simulink model "parrot_communication_host"  (R2024b)
settings: Solver=FixedStepAuto  StartTime=0.0  StopTime=inf  FixedStep=0.05  RelTol=1e-3
undefined symbols (not defined in the file or in its folder): f
libraries: instrumentlib x7
settings Model: ExtModeTrigDuration=80  Creator=The MathWorks, Inc.  LastModifiedBy=28029
settings SolverCC: AlgebraicLoopSolver=TrustRegion
settings DataIOCC: ReturnWorkspaceOutputs=off
settings OptimizationCC: DefaultParameterBehavior=Inlined  EnhancedBackFolding=on  PassReuseOutputArgsAs=Individual arguments  MaxStackSize=64  OptimizeBlockOrder=speed  DifferentSizesBufferReuse=on  OptimizationCustomize=off  EfficientTunableParamExpr=on
settings DebuggingCC: ParameterTunabilityLossMsg=error  UnconnectedInputMsg=warning  UnconnectedOutputMsg=warning  UnconnectedLineMsg=warning  ArithmeticOperatorsInVariantConditions=warning
settings HardwareCC: ProdBitPerPointer=32  ProdBitPerSizeT=32  ProdBitPerPtrDiffT=32  ProdLargestAtomicInteger=Long  ProdWordSize=32  ProdHWDeviceType=ARM Compatible->ARM 9  UseEmbeddedCoderFeatures=off  UseSimulinkCoderFeatures=off
settings ModelReferenceCC: EnableRefExpFcnMdlSchedulingChecks=on
settings SFSimCC: SimUseLocalCustomCode=off  MATLABDynamicMemAlloc=off  CustomCodeUndefinedFunction=UseInterfaceOnly
settings RTWCC: Description=Embedded Coder  SystemTargetFile=ert.tlc  TemplateMakefile=ert_default_tmf  GenerateReport=on  RTWUseLocalCustomCode=off  Toolchain=Sourcery G++ Lite GNU Toolchain for Drones  IncludeHyperlinkInReport=on  LaunchReport=on  GenerateTraceInfo=on  GenerateTraceReport=on  GenerateTraceReportSl=on  GenerateTraceReportSf=on  GenerateTraceReportEml=on  GPUComputeCapability=3.5
settings CodeAppCC: ForceParamTrailComments=on  IgnoreCustomStorageClasses=off  OperatorAnnotations=on  SimulinkDataObjDesc=on  SFDataObjDesc=on  InsertBlockDesc=on
settings ERTTargetCC: ERTCustomFileTemplate=example_file_process.tlc  DynamicArrayContainerType=coder::array

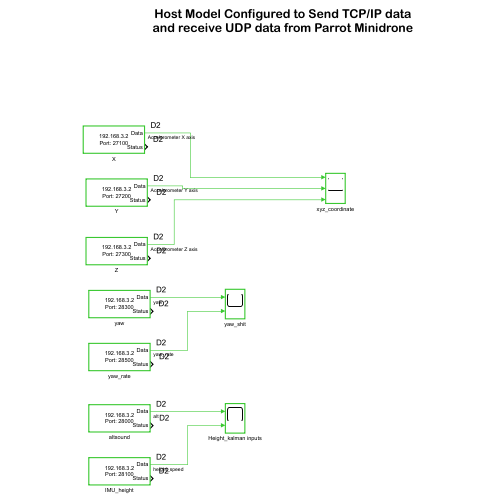
[thumbnail: Simulink's stored preview of the top-level diagram]
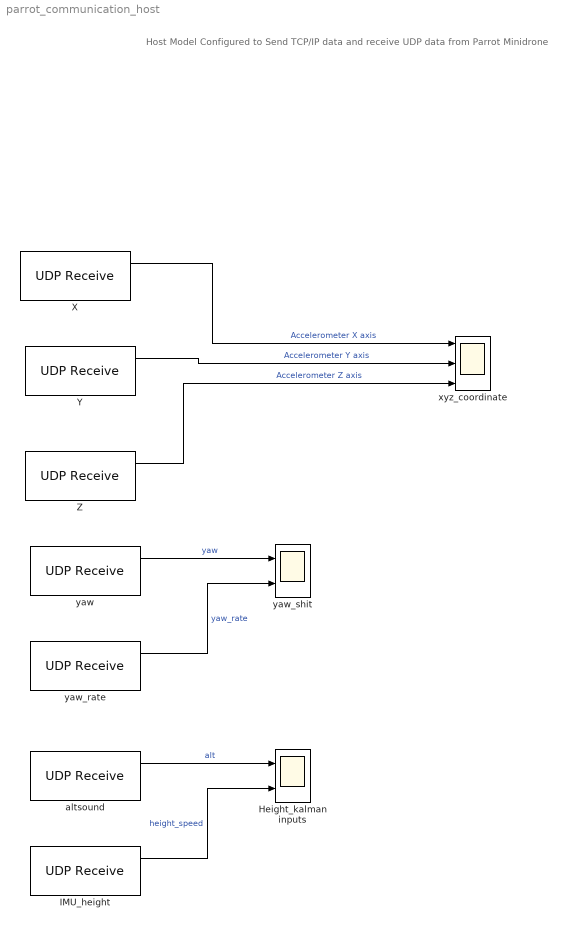
== system parrot_communication_host ==
  note: Host Model Configured to Send TCP/IP data
      | and receive UDP data from Parrot Minidrone
  Height_kalman inputs : Scope  NumInputPorts=2
  IMU_height : instrumentlib/UDP Receive  LocalAddress=192.168.3.2  LocalPort=28100  EnablePortSharing=off  Host=192.168.3.5  Port=29000  GetLatestData=off  DataSize=1  DataType=single  ASCIIFormatting=%f,  Terminator=LF  CustomTerminator=10  ByteOrder=little-endian  EnableBlockingMode=off  Timeout=10  SampleTime=1  SimulateUsing=Interpreted execution
  X : instrumentlib/UDP Receive  LocalAddress=192.168.3.2  LocalPort=27100  EnablePortSharing=off  Host=192.168.3.5  Port=29000  GetLatestData=off  DataSize=1  DataType=single  ASCIIFormatting=%f,  Terminator=LF  CustomTerminator=10  ByteOrder=little-endian  EnableBlockingMode=off  Timeout=10  SampleTime=1  SimulateUsing=Interpreted execution
  Y : instrumentlib/UDP Receive  LocalAddress=192.168.3.2  LocalPort=27200  EnablePortSharing=off  Host=192.168.3.5  Port=29000  GetLatestData=off  DataSize=1  DataType=single  ASCIIFormatting=%f,  Terminator=LF  CustomTerminator=10  ByteOrder=little-endian  EnableBlockingMode=off  Timeout=10  SampleTime=1  SimulateUsing=Interpreted execution
  Z : instrumentlib/UDP Receive  LocalAddress=192.168.3.2  LocalPort=27300  EnablePortSharing=off  Host=192.168.3.5  Port=29000  GetLatestData=off  DataSize=1  DataType=single  ASCIIFormatting=%f,  Terminator=LF  CustomTerminator=10  ByteOrder=little-endian  EnableBlockingMode=off  Timeout=10  SampleTime=1  SimulateUsing=Interpreted execution
  altsound : instrumentlib/UDP Receive  LocalAddress=192.168.3.2  LocalPort=28000  EnablePortSharing=off  Host=192.168.3.5  Port=29000  GetLatestData=off  DataSize=1  DataType=single  ASCIIFormatting=%f,  Terminator=LF  CustomTerminator=10  ByteOrder=little-endian  EnableBlockingMode=off  Timeout=10  SampleTime=1  SimulateUsing=Interpreted execution
  xyz_coordinate : Scope  NumInputPorts=3
  yaw : instrumentlib/UDP Receive  LocalAddress=192.168.3.2  LocalPort=28300  EnablePortSharing=off  Host=192.168.3.5  Port=29000  GetLatestData=off  DataSize=1  DataType=single  ASCIIFormatting=%f,  Terminator=LF  CustomTerminator=10  ByteOrder=little-endian  EnableBlockingMode=off  Timeout=10  SampleTime=1  SimulateUsing=Interpreted execution
  yaw_rate : instrumentlib/UDP Receive  LocalAddress=192.168.3.2  LocalPort=28500  EnablePortSharing=off  Host=192.168.3.5  Port=29000  GetLatestData=off  DataSize=1  DataType=single  ASCIIFormatting=%f,  Terminator=LF  CustomTerminator=10  ByteOrder=little-endian  EnableBlockingMode=off  Timeout=10  SampleTime=1  SimulateUsing=Interpreted execution
  yaw_shit : Scope  NumInputPorts=2
  wires:
  Y/1 -> xyz_coordinate/2  "Accelerometer Y axis"
  X/1 -> xyz_coordinate/1  "Accelerometer X axis"
  Z/1 -> xyz_coordinate/3  "Accelerometer Z axis"
  yaw/1 -> yaw_shit/1  "yaw"
  yaw_rate/1 -> yaw_shit/2  "yaw_rate"
  altsound/1 -> Height_kalman inputs/1  "alt"
  IMU_height/1 -> Height_kalman inputs/2  "height_speed"
